simulink model "controller"  (Simulink 8.8)
settings: Solver=FixedStepDiscrete  StartTime=0.0  StopTime=inf  FixedStep=Ts  RelTol=1e-3  EnableMultiTasking=on
InitFcn:
  | clc
  | cd(fileparts(which(bdroot)));
  | initTrqBalancingSeeSaw;
undefined symbols (not defined in the file): bVectorConstraints, CONFIG, ConstraintsMatrix, directionOfOscillation, gain, LEFT_RIGHT_FOOT_IN_CONTACT, noOscillationTime, referenceParams, reg, ROBOT_DOF, sat, seesaw, WBT_robotName
libraries: WBToolboxLibrary x51, simulink x2
settings Model: SuppressorTable=22 serialization::archive 11 0 3 0 0 0 11 0  Creator=makaveli  LastModifiedBy=gnava
settings DataIOCC: SignalLoggingSaveFormat=Dataset
settings DebuggingCC: UnderspecifiedInitializationDetection=Simplified  MergeDetectMultiDrivingBlocksExec=error  SolverPrmCheckMsg=warning  FcnCallInpInsideContextMsg=error  AllowSymbolicDim=off  StateNameClashWarn=none
settings GRTTargetCC: CombineOutputUpdateFcns=on  GRTInterface=off
settings ConfigComp: CovSFcnEnable=off

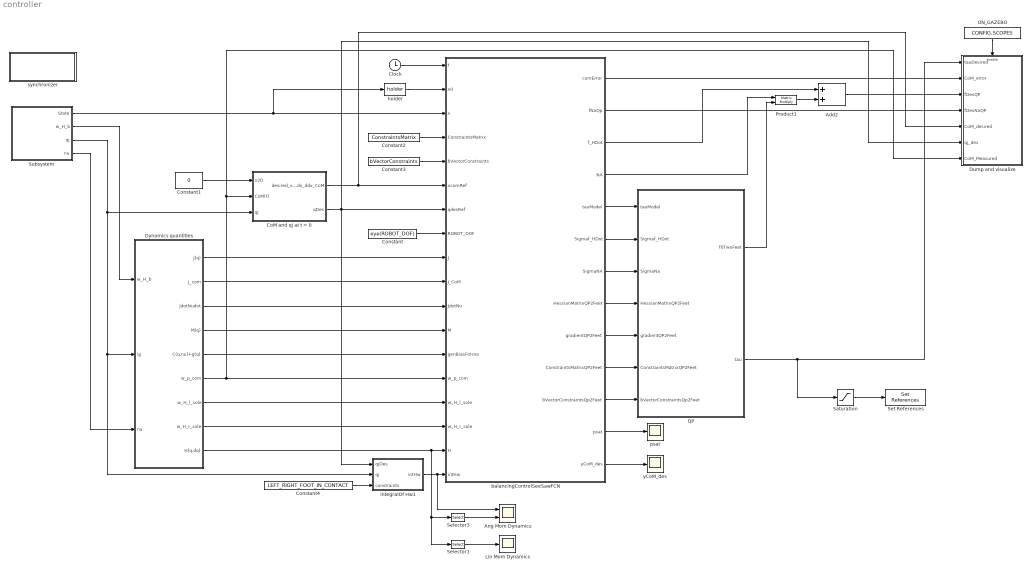
== system controller ==
  Add2 : Sum
  Ang Mom Dynamics : Scope  NumInputPorts=2
  Clock : Clock
  CoM and qj at t = 0 : Subsystem  Priority=2
  Constant : Constant  Value=eye(ROBOT_DOF)
  Constant1 : Constant  Value=0
  Constant2 : Constant  Value=ConstraintsMatrix
  Constant3 : Constant  Value=bVectorConstraints
  Constant4 : Constant  Value=LEFT_RIGHT_FOOT_IN_CONTACT
  Dump and visualize : Subsystem
  Dynamics quantities : Subsystem  Priority=3
  Lin Mom Dynamics : Scope
  "ON_GAZEBO " : Constant  Value=CONFIG.SCOPES
  Product1 : Product  Multiplication=Matrix(*)
  QP : Subsystem
  Saturation : Saturate  UpperLimit=sat.torque  LowerLimit=-sat.torque
  Selector1 : Selector  InputPortWidth=6  IndexOptions=Index vector (dialog)  Indices=[1 2 3]  OutputSizes=1
  Selector3 : Selector  InputPortWidth=6  IndexOptions=Index vector (dialog)  Indices=[4 5 6]  OutputSizes=1
  Set References : WBToolboxLibrary/wholeBodyActuators/Set References  controlType=Torque  fullOrSubControl=Full  controlledJoints=''  robotName=WBT_robotName  localName=WBT_modelName  wbiFile=WBT_wbiFilename  wbiList=WBT_wbiList
  Subsystem : Subsystem  Priority=1
      mask Display:
      | disp('State');
      | port_label('output',1,'x')
      | port_label('output',2,'w_H_b')
      | port_label('output',3,'q_j')
      | port_label('output',4,'nu')
  balancingControlSeeSawFCN : MATLAB Function  TreatAsAtomicUnit=on
  "holder " : WBToolboxLibrary/Utilities/holder 
  integralOf Hw1 : Subsystem
  psat : Scope
  synchronizer : Subsystem
      mask Display: disp('SYNCHRONIZER')
  yCoM_des : Scope
  wires:
  Clock/1 -> balancingControlSeeSawFCN/1(t)
  Subsystem/1(State) -> balancingControlSeeSawFCN/3(x), "holder "/1
  Subsystem/4(nu) -> Dynamics quantities/3(nu)
  CoM and qj at t = 0/2(qDes) -> integralOf Hw1/1(qjDes), Dump and visualize/6(qj_des), balancingControlSeeSawFCN/7(qdesRef)
  Constant/1 -> balancingControlSeeSawFCN/8(ROBOT_DOF)
  Dynamics quantities/1("J(q) ") -> balancingControlSeeSawFCN/9(J)
  Dynamics quantities/2(J_com) -> balancingControlSeeSawFCN/10(J_CoM)
  Dynamics quantities/3(JdotNudot) -> balancingControlSeeSawFCN/11(JdotNu)
  Dynamics quantities/4(M(q)) -> balancingControlSeeSawFCN/12(M)
  Dynamics quantities/5(C(q,nu)+g(q)) -> balancingControlSeeSawFCN/13(genBiasForces)
  Dynamics quantities/6(w_p_com) -> balancingControlSeeSawFCN/14(w_p_com), CoM and qj at t = 0/2(CoM(t)), Dump and visualize/7(CoM_Measured)
  Dynamics quantities/7(w_H_l_sole) -> balancingControlSeeSawFCN/15(w_H_l_sole)
  Dynamics quantities/8(w_H_r_sole) -> balancingControlSeeSawFCN/16(w_H_r_sole)
  Dynamics quantities/9(H(q,dq)) -> Selector1/1, Selector3/1, balancingControlSeeSawFCN/17(H)
  Saturation/1 -> Set References/1
  "holder "/1 -> balancingControlSeeSawFCN/2(x0)
  Subsystem/2(w_H_b) -> Dynamics quantities/1(w_H_b)
  Subsystem/3(qj) -> CoM and qj at t = 0/3(qj), integralOf Hw1/2(qj), Dynamics quantities/2(qj)
  Constant1/1 -> CoM and qj at t = 0/1(x2D)
  Constant2/1 -> balancingControlSeeSawFCN/4(ConstraintsMatrix)
  Constant3/1 -> balancingControlSeeSawFCN/5(bVectorConstraints)
  QP/1(f0TwoFeet) -> Product1/2
  QP/2(tau) -> Dump and visualize/1(tauDesired), Saturation/1
  "ON_GAZEBO "/1 -> Dump and visualize/Enable
  CoM and qj at t = 0/1(desired_x_dx_ddx_CoM) -> Dump and visualize/5(CoM_desired), balancingControlSeeSawFCN/6(xcomRef)
  balancingControlSeeSawFCN/1(comError) -> Dump and visualize/2(CoM_error)
  balancingControlSeeSawFCN/2(fNoQp) -> Dump and visualize/4(fDesNoQP)
  Product1/1 -> Add2/2
  balancingControlSeeSawFCN/4(NA) -> Product1/1
  balancingControlSeeSawFCN/3(f_HDot) -> Add2/1
  Add2/1 -> Dump and visualize/3(fDesQP)
  integralOf Hw1/1(intHw) -> Ang Mom Dynamics/1, balancingControlSeeSawFCN/18(intHw)
  balancingControlSeeSawFCN/5(tauModel) -> QP/1(tauModel)
  balancingControlSeeSawFCN/6(Sigmaf_HDot) -> QP/2(Sigmaf_HDot)
  balancingControlSeeSawFCN/7(SigmaNA) -> QP/3(SigmaNa)
  balancingControlSeeSawFCN/8(HessianMatrixQP2Feet) -> QP/4(HessianMatrixQP2Feet)
  balancingControlSeeSawFCN/9(gradientQP2Feet) -> QP/5(gradientQP2Feet)
  balancingControlSeeSawFCN/10(ConstraintsMatrixQP2Feet) -> QP/6(ConstraintsMatrixQP2Feet)
  balancingControlSeeSawFCN/11(bVectorConstraintsQp2Feet) -> QP/7(bVectorConstraintsQp2Feet)
  balancingControlSeeSawFCN/12(psat) -> psat/1
  balancingControlSeeSawFCN/13(yCoM_des) -> yCoM_des/1
  Constant4/1 -> integralOf Hw1/3(constraints)
  Selector3/1 -> Ang Mom Dynamics/2
  Selector1/1 -> Lin Mom Dynamics/1

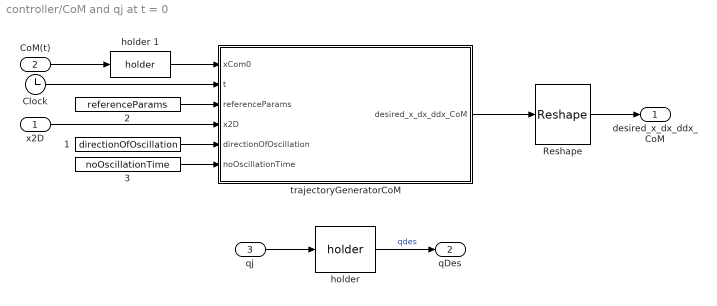
== system controller/CoM and qj at t = 0 ==
  x2D : Inport
  CoM(t) : Inport  Port=2
  qj : Inport  Port=3
  "    1" : Constant  Value=directionOfOscillation
  "    2" : Constant  Value=referenceParams
  "    3" : Constant  Value=noOscillationTime
  Clock : Clock
  Reshape : Reshape  OutputDimensionality=Customize  OutputDimensions=[3,3]
  "holder " : WBToolboxLibrary/Utilities/holder 
  holder 1 : WBToolboxLibrary/Utilities/holder 
  trajectoryGeneratorCoM : MATLAB Function  TreatAsAtomicUnit=on
  desired_x_dx_ddx_CoM : Outport
  qDes : Outport  Port=2
  wires:
  qj/1 -> "holder "/1
  "holder "/1 -> qDes/1  "qdes"
  holder 1/1 -> trajectoryGeneratorCoM/1(xCom0)
  "    2"/1 -> trajectoryGeneratorCoM/3(referenceParams)
  Clock/1 -> trajectoryGeneratorCoM/2(t)
  "    1"/1 -> trajectoryGeneratorCoM/5(directionOfOscillation)
  "    3"/1 -> trajectoryGeneratorCoM/6(noOscillationTime)
  trajectoryGeneratorCoM/1(desired_x_dx_ddx_CoM) -> Reshape/1
  Reshape/1 -> desired_x_dx_ddx_CoM/1
  x2D/1 -> trajectoryGeneratorCoM/4(x2D)
  CoM(t)/1 -> holder 1/1

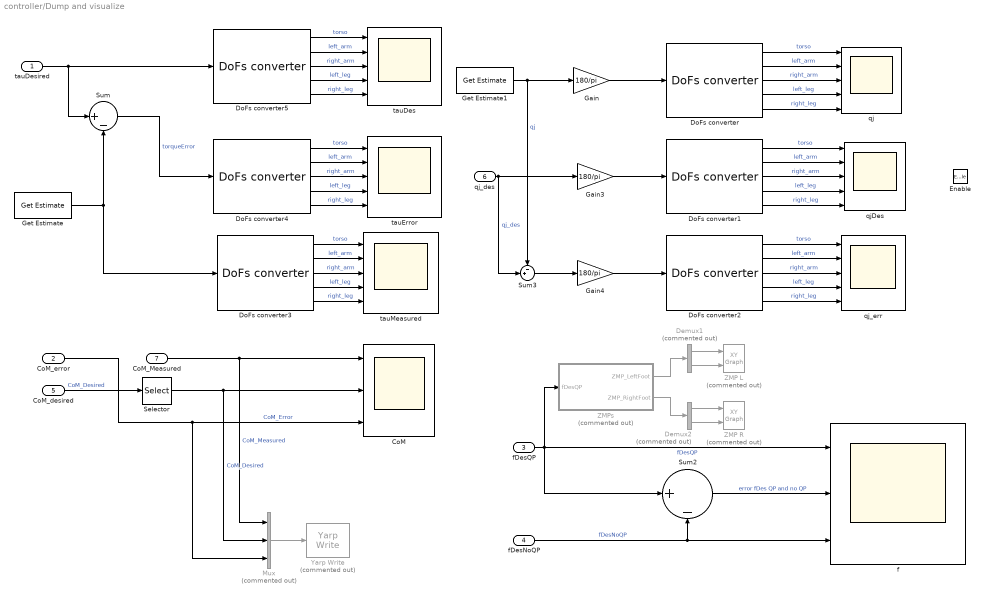
== system controller/Dump and visualize ==
  tauDesired : Inport
  CoM_error : Inport  Port=2
  fDesQP : Inport  Port=3
  fDesNoQP : Inport  Port=4
  CoM_desired : Inport  Port=5
  qj_des : Inport  Port=6
  CoM_Measured : Inport  Port=7
  Enable : EnablePort
  CoM : Scope  NumInputPorts=3
  Demux1 : Demux  Commented=on  Outputs=2
  Demux2 : Demux  Commented=on  Outputs=2
  DoFs converter{,1..5} (6 alike) : WBToolboxLibrary/Utilities/DoFs converter  yarp2WBIOption=From WBI to YARP  robotName=WBT_robotName  localName=WBT_modelName  wbiFile=WBT_wbiFilename  wbiList=WBT_wbiList
  Gain : Gain  Gain=180/pi
  Gain3 : Gain  Gain=180/pi
  Gain4 : Gain  Gain=180/pi
  Get Estimate : WBToolboxLibrary/wholeBodyStates/Get Estimate  estimateType=Joints Torque  robotName=WBT_robotName  localName=WBT_modelName  wbiFile=WBT_wbiFilename  wbiList=WBT_wbiList
  Get Estimate1 : WBToolboxLibrary/wholeBodyStates/Get Estimate  estimateType=Joints Position  robotName=WBT_robotName  localName=WBT_modelName  wbiFile=WBT_wbiFilename  wbiList=WBT_wbiList
  Mux : Mux  Commented=on  Inputs=3
  Selector : Selector  NumberOfDimensions=2  IndexOptions=Index vector (dialog),Index vector (dialog)  Indices=[1:3],1  OutputSizes=1,1
  Sum : Sum  Inputs=|+-
  Sum2 : Sum  Inputs=|+-
  Sum3 : Sum  Inputs=-+|
  Yarp Write : WBToolboxLibrary/Utilities/Yarp Write  Commented=on  portName='/oneFootBalancing/comInfo:o'  autoconnect=off  errorOnConnection=on
  ZMP L : simulink/Sinks/XY Graph  Commented=on  xmin=gain.footSize(1,1)  xmax=gain.footSize(1,2)  ymin=gain.footSize(2,1)  ymax=gain.footSize(2,2)  st=-1
  ZMP R : simulink/Sinks/XY Graph  Commented=on  xmin=gain.footSize(1,1)  xmax=gain.footSize(1,2)  ymin=gain.footSize(2,1)  ymax=gain.footSize(2,2)  st=-1
  ZMPs : Subsystem  Commented=on
  f : Scope  NumInputPorts=3
  qj : Scope  NumInputPorts=5
  qjDes : Scope  NumInputPorts=5
  qj_err : Scope  NumInputPorts=5
  tauDes : Scope  NumInputPorts=5
  tauError : Scope  NumInputPorts=5
  tauMeasured : Scope  NumInputPorts=5
  wires:
  CoM_error/1 -> Mux/3, CoM/3  "CoM_Error"
  CoM_desired/1 -> Selector/1  "CoM_Desired"
  CoM_Measured/1 -> Mux/1, CoM/1  "CoM_Measured"
  Get Estimate1/1 -> Sum3/1, Gain/1  "qj"
  Gain/1 -> DoFs converter/1
  DoFs converter/5 -> qj/5  "right_leg"
  DoFs converter/1 -> qj/1  "torso"
  DoFs converter/2 -> qj/2  "left_arm"
  DoFs converter/4 -> qj/4  "left_leg"
  DoFs converter/3 -> qj/3  "right_arm"
  fDesQP/1 -> ZMPs/1(fDesQP), Sum2/1, f/1  "fDesQP"
  ZMPs/1(ZMP_LeftFoot) -> Demux1/1
  ZMPs/2(ZMP_RightFoot) -> Demux2/1
  Demux1/1 -> ZMP L/1
  Demux1/2 -> ZMP L/2
  Demux2/1 -> ZMP R/1
  Demux2/2 -> ZMP R/2
  Sum2/1 -> f/2  "error fDes QP and no QP"
  fDesNoQP/1 -> Sum2/2, f/3  "fDesNoQP"
  tauDesired/1 -> DoFs converter5/1, Sum/1
  Get Estimate/1 -> DoFs converter3/1, Sum/2
  DoFs converter5/5 -> tauDes/5  "right_leg"
  DoFs converter5/1 -> tauDes/1  "torso"
  DoFs converter5/2 -> tauDes/2  "left_arm"
  DoFs converter5/4 -> tauDes/4  "left_leg"
  DoFs converter5/3 -> tauDes/3  "right_arm"
  DoFs converter4/5 -> tauError/5  "right_leg"
  DoFs converter4/1 -> tauError/1  "torso"
  DoFs converter4/2 -> tauError/2  "left_arm"
  DoFs converter4/4 -> tauError/4  "left_leg"
  DoFs converter4/3 -> tauError/3  "right_arm"
  Sum/1 -> DoFs converter4/1  "torqueError"
  DoFs converter3/5 -> tauMeasured/5  "right_leg"
  DoFs converter3/1 -> tauMeasured/1  "torso"
  DoFs converter3/2 -> tauMeasured/2  "left_arm"
  DoFs converter3/4 -> tauMeasured/4  "left_leg"
  DoFs converter3/3 -> tauMeasured/3  "right_arm"
  qj_des/1 -> Sum3/2, Gain3/1  "qj_des"
  Gain3/1 -> DoFs converter1/1
  DoFs converter1/5 -> qjDes/5  "right_leg"
  DoFs converter1/1 -> qjDes/1  "torso"
  DoFs converter1/2 -> qjDes/2  "left_arm"
  DoFs converter1/4 -> qjDes/4  "left_leg"
  DoFs converter1/3 -> qjDes/3  "right_arm"
  Gain4/1 -> DoFs converter2/1
  DoFs converter2/5 -> qj_err/5  "right_leg"
  DoFs converter2/1 -> qj_err/1  "torso"
  DoFs converter2/2 -> qj_err/2  "left_arm"
  DoFs converter2/4 -> qj_err/4  "left_leg"
  DoFs converter2/3 -> qj_err/3  "right_arm"
  Sum3/1 -> Gain4/1
  Selector/1 -> Mux/2, CoM/2  "CoM_Desired"
  Mux/1 -> Yarp Write/1

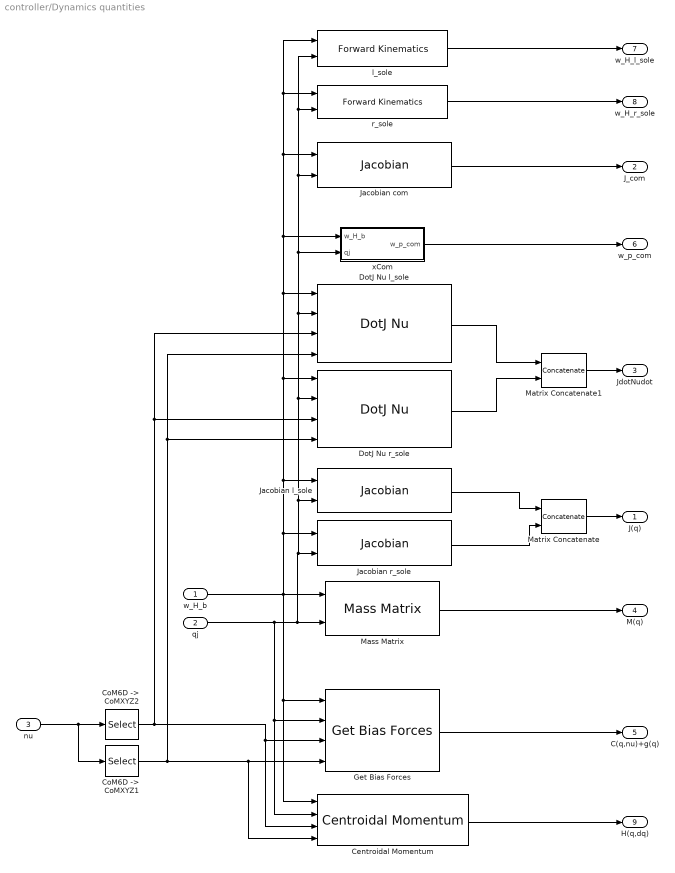
== system controller/Dynamics quantities ==
  w_H_b : Inport
  qj : Inport  Port=2
  nu : Inport  Port=3
  Centroidal Momentum : WBToolboxLibrary/wholeBodyModel/Dynamics/Centroidal Momentum  robotName=WBT_robotName  localName=WBT_modelName  wbiFile=WBT_wbiFilename  wbiList=WBT_wbiList
  "CoM6D ->  CoMXYZ1" : Selector  InputPortWidth=6+ROBOT_DOF  IndexOptions=Index vector (dialog)  Indices=[7:6+ROBOT_DOF]  OutputSizes=1
  "CoM6D ->  CoMXYZ2" : Selector  InputPortWidth=6+ROBOT_DOF  IndexOptions=Index vector (dialog)  Indices=[1 2 3 4 5 6]  OutputSizes=1
  "DotJ Nu l_sole " : WBToolboxLibrary/wholeBodyModel/Jacobians/DotJ Nu  frameName='l_sole'  robotName=WBT_robotName  localName=WBT_modelName  wbiFile=WBT_wbiFilename  wbiList=WBT_wbiList
  "DotJ Nu r_sole " : WBToolboxLibrary/wholeBodyModel/Jacobians/DotJ Nu  frameName='r_sole'  robotName=WBT_robotName  localName=WBT_modelName  wbiFile=WBT_wbiFilename  wbiList=WBT_wbiList
  Get Bias Forces : WBToolboxLibrary/wholeBodyModel/Dynamics/Get Bias Forces  robotName=WBT_robotName  localName=WBT_modelName  wbiFile=WBT_wbiFilename  wbiList=WBT_wbiList  explicitGravity=off
  Jacobian com : WBToolboxLibrary/wholeBodyModel/Jacobians/Jacobian  frameName='com'  robotName=WBT_robotName  localName=WBT_modelName  wbiFile=WBT_wbiFilename  wbiList=WBT_wbiList
  Jacobian l_sole : WBToolboxLibrary/wholeBodyModel/Jacobians/Jacobian  frameName='l_sole'  robotName=WBT_robotName  localName=WBT_modelName  wbiFile=WBT_wbiFilename  wbiList=WBT_wbiList
  Jacobian r_sole : WBToolboxLibrary/wholeBodyModel/Jacobians/Jacobian  frameName='r_sole'  robotName=WBT_robotName  localName=WBT_modelName  wbiFile=WBT_wbiFilename  wbiList=WBT_wbiList
  Mass Matrix : WBToolboxLibrary/wholeBodyModel/Dynamics/Mass Matrix  robotName=WBT_robotName  localName=WBT_modelName  wbiFile=WBT_wbiFilename  wbiList=WBT_wbiList
  Matrix Concatenate : Concatenate  Mode=Multidimensional array
  Matrix Concatenate1 : Concatenate  Mode=Multidimensional array
  l_sole : WBToolboxLibrary/wholeBodyModel/Kinematics/Forward Kinematics  frameName='l_sole'  robotName=WBT_robotName  localName=WBT_modelName  wbiFile=WBT_wbiFilename  wbiList=WBT_wbiList
  r_sole : WBToolboxLibrary/wholeBodyModel/Kinematics/Forward Kinematics  frameName='r_sole'  robotName=WBT_robotName  localName=WBT_modelName  wbiFile=WBT_wbiFilename  wbiList=WBT_wbiList
  xCom : Subsystem
  "J(q) " : Outport
  J_com : Outport  Port=2
  JdotNudot : Outport  Port=3
  M(q) : Outport  Port=4
  C(q,nu)+g(q) : Outport  Port=5
  w_p_com : Outport  Port=6
  w_H_l_sole : Outport  Port=7
  w_H_r_sole : Outport  Port=8
  H(q,dq) : Outport  Port=9
  wires:
  Get Bias Forces/1 -> C(q,nu)+g(q)/1
  Matrix Concatenate1/1 -> JdotNudot/1
  Jacobian r_sole/1 -> Matrix Concatenate/2
  l_sole/1 -> w_H_l_sole/1
  xCom/1(w_p_com) -> w_p_com/1
  r_sole/1 -> w_H_r_sole/1
  Matrix Concatenate/1 -> "J(q) "/1
  Jacobian l_sole/1 -> Matrix Concatenate/1
  Jacobian com/1 -> J_com/1
  w_H_b/1 -> Jacobian r_sole/1, "DotJ Nu r_sole "/1, r_sole/1, l_sole/1, Jacobian com/1, xCom/1(w_H_b), "DotJ Nu l_sole "/1, Jacobian l_sole/1, Mass Matrix/1, Centroidal Momentum/1, Get Bias Forces/1
  qj/1 -> r_sole/2, l_sole/2, Jacobian com/2, xCom/2(qj), "DotJ Nu l_sole "/2, "DotJ Nu r_sole "/2, Jacobian l_sole/2, Jacobian r_sole/2, Mass Matrix/2, Get Bias Forces/2, Centroidal Momentum/2
  "CoM6D ->  CoMXYZ2"/1 -> "DotJ Nu r_sole "/3, "DotJ Nu l_sole "/3, Centroidal Momentum/3, Get Bias Forces/3
  "CoM6D ->  CoMXYZ1"/1 -> "DotJ Nu r_sole "/4, "DotJ Nu l_sole "/4, Get Bias Forces/4, Centroidal Momentum/4
  nu/1 -> "CoM6D ->  CoMXYZ1"/1, "CoM6D ->  CoMXYZ2"/1
  Centroidal Momentum/1 -> H(q,dq)/1
  Mass Matrix/1 -> M(q)/1
  "DotJ Nu l_sole "/1 -> Matrix Concatenate1/1
  "DotJ Nu r_sole "/1 -> Matrix Concatenate1/2

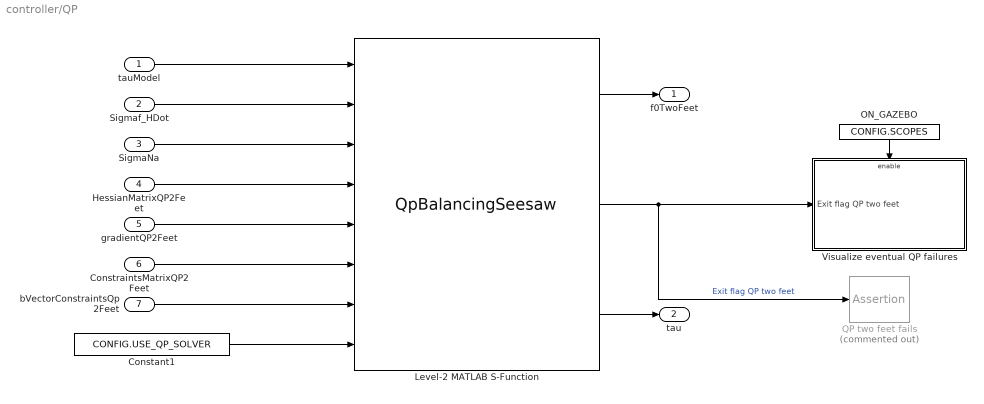
== system controller/QP ==
  tauModel : Inport
  Sigmaf_HDot : Inport  Port=2
  SigmaNa : Inport  Port=3
  HessianMatrixQP2Feet : Inport  Port=4
  gradientQP2Feet : Inport  Port=5
  ConstraintsMatrixQP2Feet : Inport  Port=6
  bVectorConstraintsQp2Feet : Inport  Port=7
  Constant1 : Constant  Value=CONFIG.USE_QP_SOLVER
  Level-2 MATLAB S-Function : M-S-Function  FunctionName=QpBalancingSeesaw
  "ON_GAZEBO " : Constant  Value=CONFIG.SCOPES
  QP two feet fails : Assertion  Commented=on
  Visualize eventual QP failures : Subsystem
  f0TwoFeet : Outport
  tau : Outport  Port=2
  wires:
  Level-2 MATLAB S-Function/1 -> f0TwoFeet/1
  Level-2 MATLAB S-Function/2 -> QP two feet fails/1, Visualize eventual QP failures/1(Exit flag QP two feet)  "Exit flag QP two feet"
  "ON_GAZEBO "/1 -> Visualize eventual QP failures/Enable
  Constant1/1 -> Level-2 MATLAB S-Function/8
  HessianMatrixQP2Feet/1 -> Level-2 MATLAB S-Function/4
  gradientQP2Feet/1 -> Level-2 MATLAB S-Function/5
  ConstraintsMatrixQP2Feet/1 -> Level-2 MATLAB S-Function/6
  bVectorConstraintsQp2Feet/1 -> Level-2 MATLAB S-Function/7
  tauModel/1 -> Level-2 MATLAB S-Function/1
  Sigmaf_HDot/1 -> Level-2 MATLAB S-Function/2
  SigmaNa/1 -> Level-2 MATLAB S-Function/3
  Level-2 MATLAB S-Function/3 -> tau/1

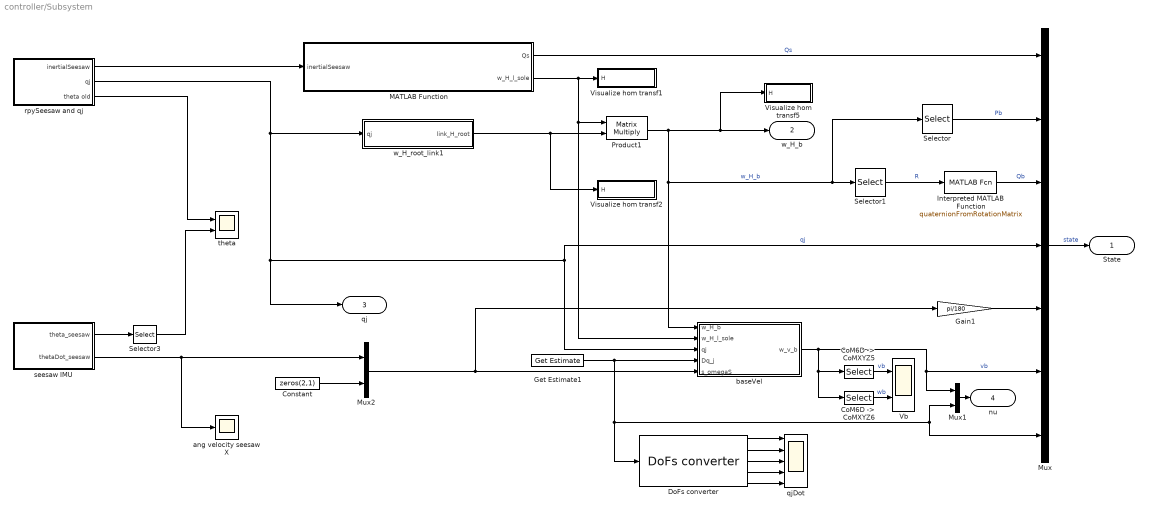
== system controller/Subsystem ==
  "CoM6D ->  CoMXYZ5" : Selector  InputPortWidth=6  IndexOptions=Index vector (dialog)  Indices=[1 2 3]  OutputSizes=1
  "CoM6D ->  CoMXYZ6" : Selector  InputPortWidth=6  IndexOptions=Index vector (dialog)  Indices=[4 5 6]  OutputSizes=1
  Constant : Constant  Value=zeros(2,1)
  DoFs converter : WBToolboxLibrary/Utilities/DoFs converter  yarp2WBIOption=From WBI to YARP  robotName=WBT_robotName  localName=WBT_modelName  wbiFile=WBT_wbiFilename  wbiList=WBT_wbiList
  Gain1 : Gain  Gain=pi/180
  Get Estimate1 : WBToolboxLibrary/wholeBodyStates/Get Estimate  estimateType=Joints Velocity  robotName=WBT_robotName  localName=WBT_modelName  wbiFile=WBT_wbiFilename  wbiList=WBT_wbiList
  Interpreted MATLAB Function : MATLABFcn  MATLABFcn=quaternionFromRotationMatrix  OutputDimensions=4
  MATLAB Function : MATLAB Function  Priority=10  TreatAsAtomicUnit=on
  Mux : Mux  Inputs=7
  Mux1 : Mux  Inputs=2
  Mux2 : Mux  Inputs=2
  Product1 : Product  Priority=19  Multiplication=Matrix(*)
  Selector : Selector  NumberOfDimensions=2  InputPortWidth=3  IndexOptions=Index vector (dialog),Index vector (dialog)  Indices=[1:3],4  OutputSizes=1,1
  Selector1 : Selector  NumberOfDimensions=2  InputPortWidth=3  IndexOptions=Index vector (dialog),Index vector (dialog)  Indices=[1:3],[1:3]  OutputSizes=1,1
  Selector3 : Selector  InputPortWidth=3  IndexOptions=Index vector (dialog)  Indices=[1]  OutputSizes=1
  "Vb " : Scope  NumInputPorts=2
  Visualize hom transf1 : Subsystem
  Visualize hom transf2 : Subsystem
  Visualize hom transf5 : Subsystem
  ang velocity seesaw X : Scope
  baseVel : Subsystem
  qjDot : Scope  NumInputPorts=5
  rpySeesaw and qj : Subsystem
  seesaw IMU : Subsystem
  theta : Scope  NumInputPorts=2
  w_H_root_link1 : Subsystem  mask{link_name='l_sole'}
      mask prompts: link_name "link name"
      mask help:
      | This block evaluates the homogeneous transformation between the world and the root link, i.e. ^wH_b. It assumes that the link specified by the variable 'link_name' has a constant position
      | w.r.t. an inertial frame, but it can rotate arbitrarily. This rotation is retrived from the IMU sensor.
      mask Display:
      | str = strrep(link_name, '_','\_');
      | port_label('output',1,['{}^{',str '}H_{root}'],'texmode','on')
      | clear str;
      | 
      | port_label('input',1,'q_j','texmode','on')
  State : Outport
  w_H_b : Outport  Port=2
  qj : Outport  Port=3
  nu : Outport  Port=4
  wires:
  Get Estimate1/1 -> baseVel/4(Dq_j), DoFs converter/1, Mux1/2, Mux/7
  rpySeesaw and qj/2(qj) -> w_H_root_link1/1(qj), qj/1, baseVel/3(qj), Mux/4  "qj"
  Mux/1 -> State/1  "state"
  Selector/1 -> Mux/2  "Pb"
  Selector1/1 -> Interpreted MATLAB Function/1  "R"
  Interpreted MATLAB Function/1 -> Mux/3  "Qb"
  Mux1/1 -> nu/1
  baseVel/1(w_v_b) -> Mux1/1, Mux/6, "CoM6D ->  CoMXYZ5"/1, "CoM6D ->  CoMXYZ6"/1  "vb"
  MATLAB Function/1(Qs) -> Mux/1  "Qs"
  Product1/1 -> Visualize hom transf5/1(H), w_H_b/1, baseVel/1(w_H_b), Selector1/1, Selector/1  "w_H_b"
  MATLAB Function/2(w_H_l_sole) -> baseVel/2(w_H_l_sole), Product1/1, Visualize hom transf1/1(H)
  w_H_root_link1/1(link_H_root) -> Visualize hom transf2/1(H), Product1/2
  DoFs converter/1 -> qjDot/1
  DoFs converter/2 -> qjDot/2
  DoFs converter/3 -> qjDot/3
  DoFs converter/4 -> qjDot/4
  DoFs converter/5 -> qjDot/5
  "CoM6D ->  CoMXYZ5"/1 -> "Vb "/1  "vb"
  "CoM6D ->  CoMXYZ6"/1 -> "Vb "/2  "wb"
  Gain1/1 -> Mux/5
  Mux2/1 -> Gain1/1, baseVel/5(s_omegaS)
  Constant/1 -> Mux2/2
  rpySeesaw and qj/1(inertialSeesaw) -> MATLAB Function/1(inertialSeesaw)
  rpySeesaw and qj/3(theta old) -> theta/1
  seesaw IMU/2(thetaDot_seesaw) -> Mux2/1, ang velocity seesaw X/1
  seesaw IMU/1(theta_seesaw) -> Selector3/1
  Selector3/1 -> theta/2

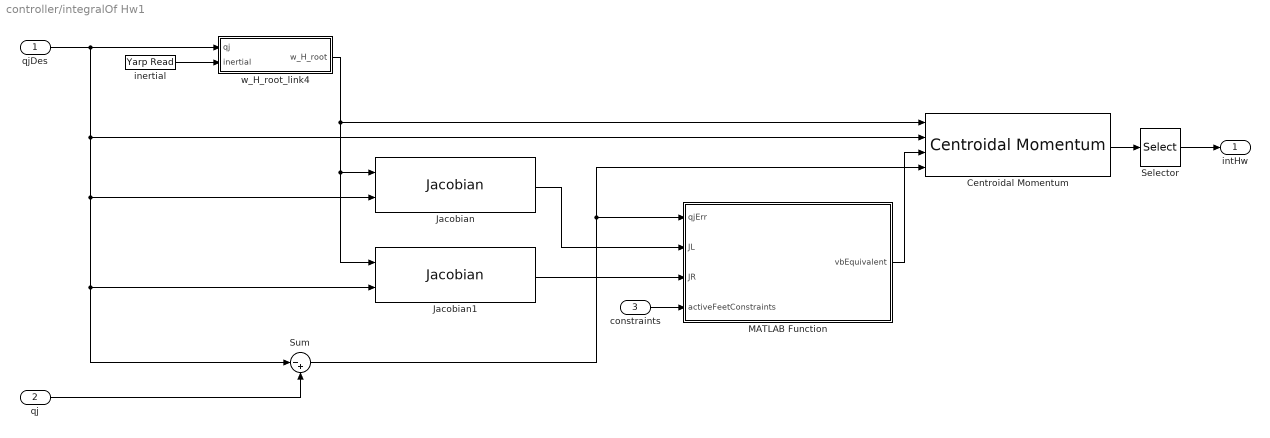
== system controller/integralOf Hw1 ==
  qjDes : Inport
  qj : Inport  Port=2
  constraints : Inport  Port=3
  Centroidal Momentum : WBToolboxLibrary/wholeBodyModel/Dynamics/Centroidal Momentum  robotName=WBT_robotName  localName=WBT_modelName  wbiFile=WBT_wbiFilename  wbiList=WBT_wbiList
  Jacobian : WBToolboxLibrary/wholeBodyModel/Jacobians/Jacobian  frameName='l_sole'  robotName=WBT_robotName  localName=WBT_modelName  wbiFile=WBT_wbiFilename  wbiList=WBT_wbiList
  Jacobian1 : WBToolboxLibrary/wholeBodyModel/Jacobians/Jacobian  frameName='r_sole'  robotName=WBT_robotName  localName=WBT_modelName  wbiFile=WBT_wbiFilename  wbiList=WBT_wbiList
  MATLAB Function : MATLAB Function  TreatAsAtomicUnit=on
  Selector : Selector  InputPortWidth=6  IndexOptions=Index vector (dialog)  Indices=[4 5 6]  OutputSizes=1
  Sum : Sum  Inputs=|-+
  inertial : WBToolboxLibrary/Utilities/Yarp Read  portName=PORTS.IMU  signalSize=12  blocking=off  timestamp=off  autoconnect=on  errorOnConnection=on
  w_H_root_link4 : Subsystem  mask{link_name='l_sole'}
      mask prompts: link_name "link name"
      mask help:
      | This block evaluates the homogeneous transformation between the world and the root link, i.e. ^wH_b. It assumes that the link specified by the variable 'link_name' has a constant position
      | w.r.t. an inertial frame, but it can rotate arbitrarily. This rotation is retrived from the IMU sensor.
      mask Display:
      | str = strrep(link_name, '_','\_');
      | port_label('output',1,['{}^{',str '}H_{root}'],'texmode','on')
      | clear str;
      | 
      | port_label('input',1,'q_j','texmode','on')
      | 
      | port_label('input',2,'inertial','texmode','on')
  intHw : Outport
  wires:
  qjDes/1 -> Sum/1, Jacobian1/2, Jacobian/2, Centroidal Momentum/2, w_H_root_link4/1(qj)
  w_H_root_link4/1(w_H_root) -> Centroidal Momentum/1, Jacobian/1, Jacobian1/1
  qj/1 -> Sum/2
  Sum/1 -> Centroidal Momentum/4, MATLAB Function/1(qjErr)
  MATLAB Function/1(vbEquivalent) -> Centroidal Momentum/3
  Jacobian/1 -> MATLAB Function/2(JL)
  Centroidal Momentum/1 -> Selector/1
  Selector/1 -> intHw/1
  Jacobian1/1 -> MATLAB Function/3(JR)
  constraints/1 -> MATLAB Function/4(activeFeetConstraints)
  inertial/1 -> w_H_root_link4/2(inertial)

== system controller/synchronizer ==
  GAZEBO_SYNCHRONIZER : Subsystem  Commented=on
  Logical Operator : Logic  Operator=NOT  AllPortsSameDT=off  OutDataTypeStr=boolean
  "ON_GAZEBO " : Constant  Value=CONFIG.ON_GAZEBO
  REAL_TIME_SYNC : Subsystem
  wires:
  Logical Operator/1 -> REAL_TIME_SYNC/Enable
  "ON_GAZEBO "/1 -> Logical Operator/1, GAZEBO_SYNCHRONIZER/Enable

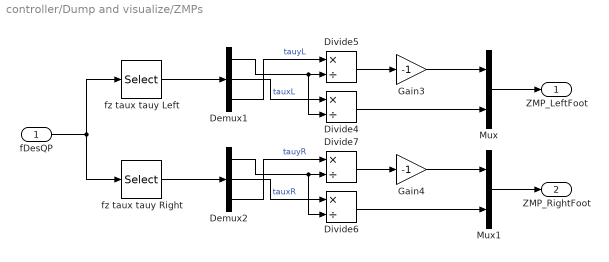
== system controller/Dump and visualize/ZMPs ==
  fDesQP : Inport
  Demux1 : Demux  Outputs=3
  Demux2 : Demux  Outputs=3
  Divide{4..7} (4 alike) : Product  Inputs=*/
  Gain3 : Gain  Gain=-1
  Gain4 : Gain  Gain=-1
  Mux : Mux  Inputs=2
  Mux1 : Mux  Inputs=2
  fz taux tauy Left : Selector  InputPortWidth=12  IndexOptions=Index vector (dialog)  Indices=[3 4 5]  OutputSizes=1
  fz taux tauy Right : Selector  InputPortWidth=12  IndexOptions=Index vector (dialog)  Indices=[9 10 11]  OutputSizes=1
  ZMP_LeftFoot : Outport
  ZMP_RightFoot : Outport  Port=2
  wires:
  fz taux tauy Left/1 -> Demux1/1
  Demux1/1 -> Divide4/2, Divide5/2
  Divide7/1 -> Gain4/1
  Divide4/1 -> Mux/2
  Divide5/1 -> Gain3/1
  fz taux tauy Right/1 -> Demux2/1
  Demux2/1 -> Divide6/2, Divide7/2
  fDesQP/1 -> fz taux tauy Left/1, fz taux tauy Right/1
  Gain3/1 -> Mux/1
  Mux/1 -> ZMP_LeftFoot/1
  Divide6/1 -> Mux1/2
  Gain4/1 -> Mux1/1
  Mux1/1 -> ZMP_RightFoot/1
  Demux1/2 -> Divide4/1  "tauxL"
  Demux1/3 -> Divide5/1  "tauyL"
  Demux2/2 -> Divide6/1  "tauxR"
  Demux2/3 -> Divide7/1  "tauyR"

== system controller/Dynamics quantities/xCom ==
  w_H_b : Inport
  qj : Inport  Port=2
  "CoM6D ->  CoMXYZ2" : Selector  NumberOfDimensions=2  InputPortWidth=7  IndexOptions=Index vector (dialog),Index vector (dialog)  Indices=[1 2 3],[4]  OutputSizes=1,1
  com : WBToolboxLibrary/wholeBodyModel/Kinematics/Forward Kinematics  frameName='com'  robotName=WBT_robotName  localName=WBT_modelName  wbiFile=WBT_wbiFilename  wbiList=WBT_wbiList
  w_p_com : Outport
  wires:
  qj/1 -> com/2
  "CoM6D ->  CoMXYZ2"/1 -> w_p_com/1
  com/1 -> "CoM6D ->  CoMXYZ2"/1
  w_H_b/1 -> com/1

== system controller/QP/Visualize eventual QP failures ==
  Exit flag QP two feet : Inport
  Enable : EnablePort
  "QP status (0: no failure, 1: not using)" : Scope
  wires:
  Exit flag QP two feet/1 -> "QP status (0: no failure, 1: not using)"/1  "Exit flag QP two feet"

== system controller/Subsystem/Visualize hom transf1 ==
  H : Inport
  "CoM6D ->  CoMXYZ1" : Selector  NumberOfDimensions=2  InputPortWidth=7  IndexOptions=Index vector (dialog),Index vector (dialog)  Indices=[1 2 3],[1 2 3]  OutputSizes=1,1
  Hom : Scope
  MATLAB Function : MATLAB Function  TreatAsAtomicUnit=on
  p : Scope
  position : Selector  NumberOfDimensions=2  InputPortWidth=7  IndexOptions=Index vector (dialog),Index vector (dialog)  Indices=[1 2 3],[4]  OutputSizes=1,1
  rollPitchYaw : Scope
  wires:
  position/1 -> p/1  "position"
  H/1 -> position/1, Hom/1, "CoM6D ->  CoMXYZ1"/1  "H"
  "CoM6D ->  CoMXYZ1"/1 -> MATLAB Function/1(R)
  MATLAB Function/1(rollPitchYaw) -> rollPitchYaw/1  "rollPitchYaw"

== system controller/Subsystem/Visualize hom transf2 ==
  H : Inport
  "CoM6D ->  CoMXYZ1" : Selector  NumberOfDimensions=2  InputPortWidth=7  IndexOptions=Index vector (dialog),Index vector (dialog)  Indices=[1 2 3],[1 2 3]  OutputSizes=1,1
  Hom : Scope
  MATLAB Function : MATLAB Function  TreatAsAtomicUnit=on
  p : Scope
  position : Selector  NumberOfDimensions=2  InputPortWidth=7  IndexOptions=Index vector (dialog),Index vector (dialog)  Indices=[1 2 3],[4]  OutputSizes=1,1
  rollPitchYaw : Scope
  wires:
  position/1 -> p/1  "position"
  H/1 -> position/1, Hom/1, "CoM6D ->  CoMXYZ1"/1  "H"
  "CoM6D ->  CoMXYZ1"/1 -> MATLAB Function/1(R)
  MATLAB Function/1(rollPitchYaw) -> rollPitchYaw/1  "rollPitchYaw"

== system controller/Subsystem/Visualize hom transf5 ==
  H : Inport
  "CoM6D ->  CoMXYZ1" : Selector  NumberOfDimensions=2  InputPortWidth=7  IndexOptions=Index vector (dialog),Index vector (dialog)  Indices=[1 2 3],[1 2 3]  OutputSizes=1,1
  Hom : Scope
  MATLAB Function : MATLAB Function  TreatAsAtomicUnit=on
  p : Scope
  position : Selector  NumberOfDimensions=2  InputPortWidth=7  IndexOptions=Index vector (dialog),Index vector (dialog)  Indices=[1 2 3],[4]  OutputSizes=1,1
  rollPitchYaw : Scope
  wires:
  position/1 -> p/1  "position"
  H/1 -> position/1, Hom/1, "CoM6D ->  CoMXYZ1"/1  "H"
  "CoM6D ->  CoMXYZ1"/1 -> MATLAB Function/1(R)
  MATLAB Function/1(rollPitchYaw) -> rollPitchYaw/1  "rollPitchYaw"

== system controller/Subsystem/baseVel ==
  w_H_b : Inport
  w_H_l_sole : Inport  Port=2
  qj : Inport  Port=3
  Dq_j : Inport  Port=4
  s_omegaS : Inport  Port=5
  Jacobian l_sole : WBToolboxLibrary/wholeBodyModel/Jacobians/Jacobian  frameName='l_sole'  robotName=WBT_robotName  localName=WBT_modelName  wbiFile=WBT_wbiFilename  wbiList=WBT_wbiList
  evaluateBaseVelocity : MATLAB Function  Priority=10  TreatAsAtomicUnit=on
  w_v_b : Outport
  wires:
  w_H_l_sole/1 -> evaluateBaseVelocity/2(w_H_l_sole)
  w_H_b/1 -> Jacobian l_sole/1
  evaluateBaseVelocity/1(w_v_base) -> w_v_b/1
  s_omegaS/1 -> evaluateBaseVelocity/4(s_omega_s)
  qj/1 -> Jacobian l_sole/2
  Dq_j/1 -> evaluateBaseVelocity/3(dq_j)
  Jacobian l_sole/1 -> evaluateBaseVelocity/1(J_l_sole)

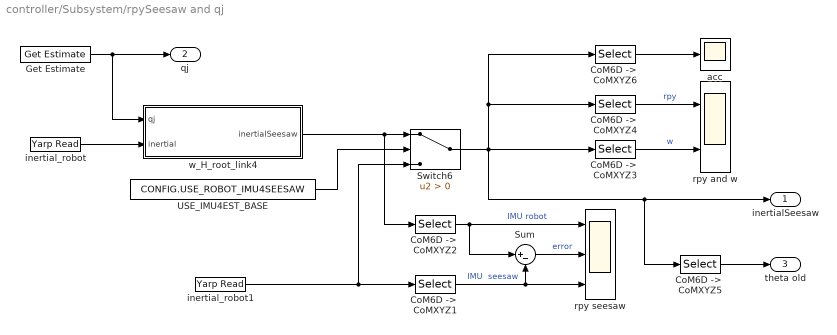
== system controller/Subsystem/rpySeesaw and qj ==
  "CoM6D ->  CoMXYZ1" : Selector  InputPortWidth=12  IndexOptions=Index vector (dialog)  Indices=[1 2 3]  OutputSizes=1
  "CoM6D ->  CoMXYZ2" : Selector  InputPortWidth=12  IndexOptions=Index vector (dialog)  Indices=[1 2 3]  OutputSizes=1
  "CoM6D ->  CoMXYZ3" : Selector  InputPortWidth=12  IndexOptions=Index vector (dialog)  Indices=[7 8 9]  OutputSizes=1
  "CoM6D ->  CoMXYZ4" : Selector  InputPortWidth=12  IndexOptions=Index vector (dialog)  Indices=[1 2 3]  OutputSizes=1
  "CoM6D ->  CoMXYZ5" : Selector  InputPortWidth=12  IndexOptions=Index vector (dialog)  Indices=[1]  OutputSizes=1
  "CoM6D ->  CoMXYZ6" : Selector  InputPortWidth=12  IndexOptions=Index vector (dialog)  Indices=[4 5 6]  OutputSizes=1
  Get Estimate : WBToolboxLibrary/wholeBodyStates/Get Estimate  estimateType=Joints Position  robotName=WBT_robotName  localName=WBT_modelName  wbiFile=WBT_wbiFilename  wbiList=WBT_wbiList
  Sum : Sum  Inputs=|+-
  Switch6 : Switch  Criteria=u2 > Threshold
  USE_IMU4EST_BASE : Constant  Value=CONFIG.USE_ROBOT_IMU4SEESAW
  acc : Scope
  inertial_robot : WBToolboxLibrary/Utilities/Yarp Read  portName=PORTS.IMU  signalSize=12  blocking=off  timestamp=off  autoconnect=on  errorOnConnection=on
  inertial_robot1 : WBToolboxLibrary/Utilities/Yarp Read  portName=PORTS.IMU  signalSize=12  blocking=off  timestamp=off  autoconnect=on  errorOnConnection=on
  rpy and w : Scope  NumInputPorts=2
  rpy seesaw : Scope  NumInputPorts=3
  w_H_root_link4 : Subsystem  mask{link_name='l_sole'}
      mask prompts: link_name "link name"
      mask help:
      | This block evaluates the homogeneous transformation between the world and the root link, i.e. ^wH_b. It assumes that the link specified by the variable 'link_name' has a constant position
      | w.r.t. an inertial frame, but it can rotate arbitrarily. This rotation is retrived from the IMU sensor.
      mask Display:
      | str = strrep(link_name, '_','\_');
      | port_label('output',1,'inertialSeesaw','texmode','on')
      | clear str;
      | 
      | port_label('input',1,'q_j','texmode','on')
      | 
      | port_label('input',2,'inertial','texmode','on')
  inertialSeesaw : Outport
  qj : Outport  Port=2
  theta old : Outport  Port=3
  wires:
  USE_IMU4EST_BASE/1 -> Switch6/2
  w_H_root_link4/1(inertialSeesaw) -> "CoM6D ->  CoMXYZ2"/1, Switch6/1
  Get Estimate/1 -> qj/1, w_H_root_link4/1(qj)
  inertial_robot/1 -> w_H_root_link4/2(inertial)
  "CoM6D ->  CoMXYZ2"/1 -> Sum/1, rpy seesaw/1  "IMU robot"
  Sum/1 -> rpy seesaw/2  "error"
  "CoM6D ->  CoMXYZ1"/1 -> Sum/2, rpy seesaw/3  "IMU  seesaw"
  "CoM6D ->  CoMXYZ3"/1 -> rpy and w/2  "w"
  "CoM6D ->  CoMXYZ4"/1 -> rpy and w/1  "rpy"
  "CoM6D ->  CoMXYZ5"/1 -> theta old/1
  inertial_robot1/1 -> Switch6/3, "CoM6D ->  CoMXYZ1"/1
  Switch6/1 -> "CoM6D ->  CoMXYZ6"/1, "CoM6D ->  CoMXYZ4"/1, "CoM6D ->  CoMXYZ3"/1, "CoM6D ->  CoMXYZ5"/1, inertialSeesaw/1
  "CoM6D ->  CoMXYZ6"/1 -> acc/1

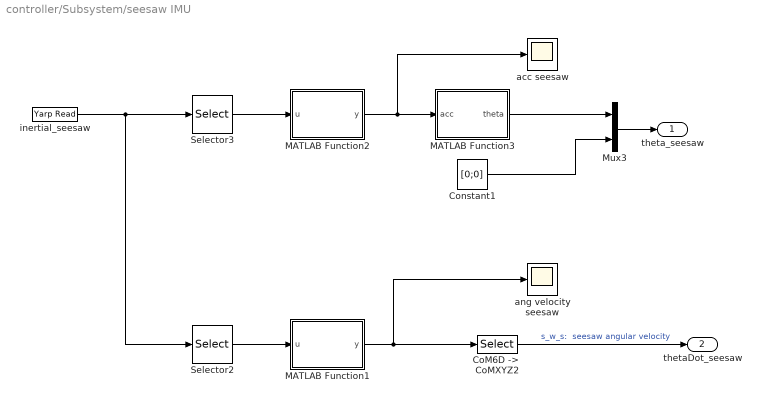
== system controller/Subsystem/seesaw IMU ==
  "CoM6D ->  CoMXYZ2" : Selector  InputPortWidth=3  IndexOptions=Index vector (dialog)  Indices=[1]  OutputSizes=1
  Constant1 : Constant  Value=[0;0]
  MATLAB Function1 : MATLAB Function  TreatAsAtomicUnit=on
  MATLAB Function2 : MATLAB Function  TreatAsAtomicUnit=on
  MATLAB Function3 : MATLAB Function  TreatAsAtomicUnit=on
  Mux3 : Mux  Inputs=2
  Selector2 : Selector  InputPortWidth=9  IndexOptions=Index vector (dialog)  Indices=[7 8 9]  OutputSizes=1
  Selector3 : Selector  InputPortWidth=9  IndexOptions=Index vector (dialog)  Indices=[4 5 6]  OutputSizes=1
  acc seesaw : Scope
  ang velocity seesaw : Scope
  inertial_seesaw : WBToolboxLibrary/Utilities/Yarp Read  portName='/seesaw'  signalSize=9  blocking=off  timestamp=off  autoconnect=on  errorOnConnection=on
  theta_seesaw : Outport
  thetaDot_seesaw : Outport  Port=2
  wires:
  Constant1/1 -> Mux3/2
  "CoM6D ->  CoMXYZ2"/1 -> thetaDot_seesaw/1  "s_w_s:  seesaw angular velocity"
  MATLAB Function2/1(y) -> acc seesaw/1, MATLAB Function3/1(acc)
  Selector3/1 -> MATLAB Function2/1(u)
  Selector2/1 -> MATLAB Function1/1(u)
  MATLAB Function3/1(theta) -> Mux3/1
  MATLAB Function1/1(y) -> ang velocity seesaw/1, "CoM6D ->  CoMXYZ2"/1
  inertial_seesaw/1 -> Selector3/1, Selector2/1
  Mux3/1 -> theta_seesaw/1

== system controller/Subsystem/w_H_root_link1 ==
  qj : Inport
  Constant2 : Constant  Value=eye(4)
  Constant6 : Constant  Value=eye(4)
  Inv\*1 : Product  Inputs=/*  Multiplication=Matrix(*)
  link : WBToolboxLibrary/wholeBodyModel/Kinematics/Forward Kinematics  frameName=link_name  robotName=WBT_robotName  localName=WBT_modelName  wbiFile=WBT_wbiFilename  wbiList=WBT_wbiList
  root_link : WBToolboxLibrary/wholeBodyModel/Kinematics/Forward Kinematics  frameName='root_link'  robotName=WBT_robotName  localName=WBT_modelName  wbiFile=WBT_wbiFilename  wbiList=WBT_wbiList
  link_H_root : Outport
  wires:
  Constant6/1 -> link/1
  Inv\*1/1 -> link_H_root/1  "link_H_root"
  link/1 -> Inv\*1/1
  Constant2/1 -> root_link/1
  qj/1 -> root_link/2, link/2
  root_link/1 -> Inv\*1/2

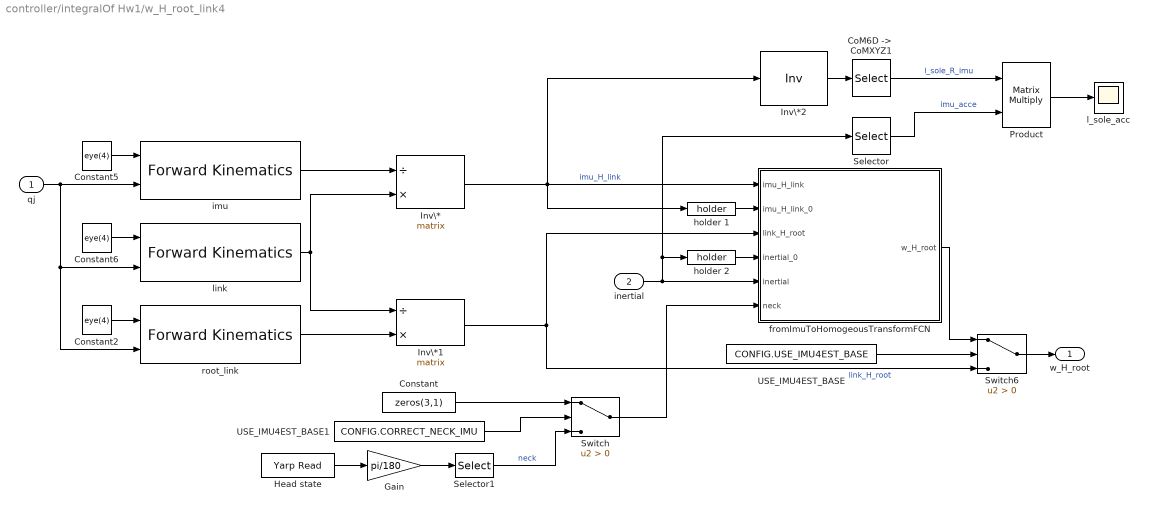
== system controller/integralOf Hw1/w_H_root_link4 ==
  qj : Inport
  inertial : Inport  Port=2
  "CoM6D ->  CoMXYZ1" : Selector  NumberOfDimensions=2  InputPortWidth=7  IndexOptions=Index vector (dialog),Index vector (dialog)  Indices=[1 2 3],[1 2 3]  OutputSizes=1,1
  Constant : Constant  Value=zeros(3,1)
  Constant2 : Constant  Value=eye(4)
  Constant5 : Constant  Value=eye(4)
  Constant6 : Constant  Value=eye(4)
  Gain : Gain  Gain=pi/180
  Head state : WBToolboxLibrary/Utilities/Yarp Read  portName=[WBT_robotName, '/head/state:o']  signalSize=6  blocking=off  timestamp=off  autoconnect=on  errorOnConnection=off
  Inv\* : Product  Inputs=/*  Multiplication=Matrix(*)
  Inv\*1 : Product  Inputs=/*  Multiplication=Matrix(*)
  Inv\*2 : Product  Inputs=/  Multiplication=Matrix(*)
  Product : Product  Multiplication=Matrix(*)
  Selector : Selector  InputPortWidth=12  IndexOptions=Index vector (dialog)  Indices=[4 5 6 ]  OutputSizes=1
  Selector1 : Selector  InputPortWidth=6  IndexOptions=Index vector (dialog)  Indices=[1:3]  OutputSizes=1
  Switch : Switch  Criteria=u2 > Threshold
  Switch6 : Switch  Criteria=u2 > Threshold
  USE_IMU4EST_BASE : Constant  Value=CONFIG.USE_IMU4EST_BASE
  USE_IMU4EST_BASE1 : Constant  Value=CONFIG.CORRECT_NECK_IMU
  fromImuToHomogeousTransformFCN : MATLAB Function  TreatAsAtomicUnit=on
  holder 1 : WBToolboxLibrary/Utilities/holder 
  holder 2 : WBToolboxLibrary/Utilities/holder 
  imu : WBToolboxLibrary/wholeBodyModel/Kinematics/Forward Kinematics  frameName='imu_frame'  robotName=WBT_robotName  localName=WBT_modelName  wbiFile=WBT_wbiFilename  wbiList=WBT_wbiList
  l_sole_acc : Scope
  link : WBToolboxLibrary/wholeBodyModel/Kinematics/Forward Kinematics  frameName=link_name  robotName=WBT_robotName  localName=WBT_modelName  wbiFile=WBT_wbiFilename  wbiList=WBT_wbiList
  root_link : WBToolboxLibrary/wholeBodyModel/Kinematics/Forward Kinematics  frameName='root_link'  robotName=WBT_robotName  localName=WBT_modelName  wbiFile=WBT_wbiFilename  wbiList=WBT_wbiList
  w_H_root : Outport
  wires:
  Constant5/1 -> imu/1
  Inv\*/1 -> Inv\*2/1, holder 1/1, fromImuToHomogeousTransformFCN/1(imu_H_link)  "imu_H_link"
  imu/1 -> Inv\*/1
  Constant6/1 -> link/1
  Inv\*1/1 -> Switch6/3, fromImuToHomogeousTransformFCN/3(link_H_root)  "link_H_root"
  link/1 -> Inv\*/2, Inv\*1/1
  inertial/1 -> Selector/1, holder 2/1, fromImuToHomogeousTransformFCN/5(inertial)
  Switch6/1 -> w_H_root/1
  USE_IMU4EST_BASE/1 -> Switch6/2
  fromImuToHomogeousTransformFCN/1(w_H_root) -> Switch6/1
  Constant2/1 -> root_link/1
  qj/1 -> root_link/2, link/2, imu/2
  root_link/1 -> Inv\*1/2
  holder 1/1 -> fromImuToHomogeousTransformFCN/2(imu_H_link_0)
  holder 2/1 -> fromImuToHomogeousTransformFCN/4(inertial_0)
  Inv\*2/1 -> "CoM6D ->  CoMXYZ1"/1
  "CoM6D ->  CoMXYZ1"/1 -> Product/1  "l_sole_R_imu"
  Selector/1 -> Product/2  "imu_acce"
  Product/1 -> l_sole_acc/1
  Head state/1 -> Gain/1
  Selector1/1 -> Switch/3  "neck"
  Constant/1 -> Switch/1
  USE_IMU4EST_BASE1/1 -> Switch/2
  Switch/1 -> fromImuToHomogeousTransformFCN/6(neck)
  Gain/1 -> Selector1/1

== system controller/synchronizer/GAZEBO_SYNCHRONIZER ==
  Enable : EnablePort
  Simulator Synchronizer : WBToolboxLibrary/Utilities/Simulator Synchronizer  period=CONFIG.TS  serverPortName='/clock/rpc'  clientPortName='/WBT_synchronizer/rpc:o'

== system controller/synchronizer/REAL_TIME_SYNC ==
  Enable : EnablePort
  Real Time Synchronizer : WBToolboxLibrary/Utilities/Real Time Synchronizer  period=CONFIG.TS

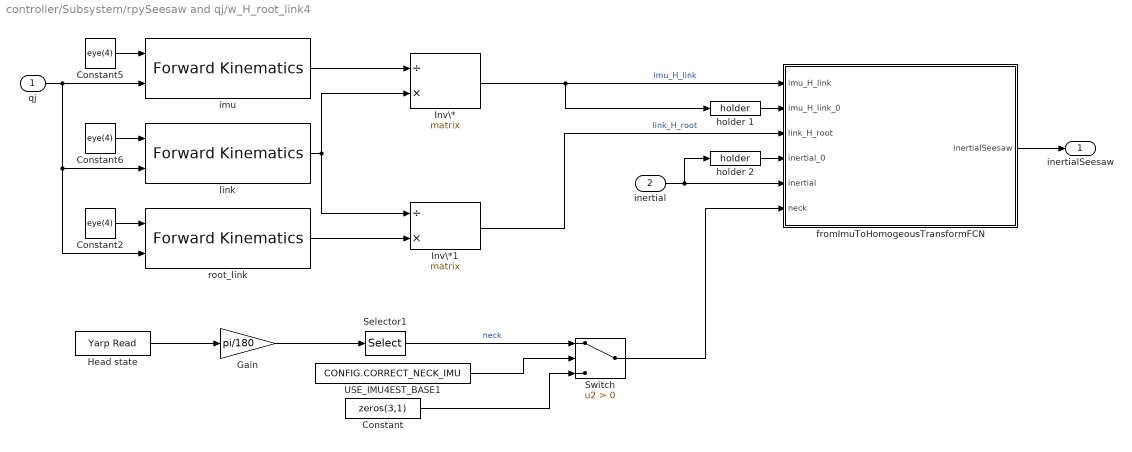
== system controller/Subsystem/rpySeesaw and qj/w_H_root_link4 ==
  qj : Inport
  inertial : Inport  Port=2
  Constant : Constant  Value=zeros(3,1)
  Constant2 : Constant  Value=eye(4)
  Constant5 : Constant  Value=eye(4)
  Constant6 : Constant  Value=eye(4)
  Gain : Gain  Gain=pi/180
  Head state : WBToolboxLibrary/Utilities/Yarp Read  portName=PORTS.NECK  signalSize=6  blocking=off  timestamp=off  autoconnect=on  errorOnConnection=on
  Inv\* : Product  Inputs=/*  Multiplication=Matrix(*)
  Inv\*1 : Product  Inputs=/*  Multiplication=Matrix(*)
  Selector1 : Selector  InputPortWidth=6  IndexOptions=Index vector (dialog)  Indices=[1:3]  OutputSizes=1
  Switch : Switch  Criteria=u2 > Threshold
  USE_IMU4EST_BASE1 : Constant  Value=CONFIG.CORRECT_NECK_IMU
  fromImuToHomogeousTransformFCN : MATLAB Function  TreatAsAtomicUnit=on
  holder 1 : WBToolboxLibrary/Utilities/holder 
  holder 2 : WBToolboxLibrary/Utilities/holder 
  imu : WBToolboxLibrary/wholeBodyModel/Kinematics/Forward Kinematics  frameName='imu_frame'  robotName=WBT_robotName  localName=WBT_modelName  wbiFile=WBT_wbiFilename  wbiList=WBT_wbiList
  link : WBToolboxLibrary/wholeBodyModel/Kinematics/Forward Kinematics  frameName=link_name  robotName=WBT_robotName  localName=WBT_modelName  wbiFile=WBT_wbiFilename  wbiList=WBT_wbiList
  root_link : WBToolboxLibrary/wholeBodyModel/Kinematics/Forward Kinematics  frameName='root_link'  robotName=WBT_robotName  localName=WBT_modelName  wbiFile=WBT_wbiFilename  wbiList=WBT_wbiList
  inertialSeesaw : Outport
  wires:
  Constant5/1 -> imu/1
  Inv\*/1 -> holder 1/1, fromImuToHomogeousTransformFCN/1(imu_H_link)  "imu_H_link"
  imu/1 -> Inv\*/1
  Constant6/1 -> link/1
  Inv\*1/1 -> fromImuToHomogeousTransformFCN/3(link_H_root)  "link_H_root"
  link/1 -> Inv\*/2, Inv\*1/1
  inertial/1 -> holder 2/1, fromImuToHomogeousTransformFCN/5(inertial)
  fromImuToHomogeousTransformFCN/1(inertialSeesaw) -> inertialSeesaw/1
  Constant2/1 -> root_link/1
  qj/1 -> root_link/2, link/2, imu/2
  root_link/1 -> Inv\*1/2
  holder 1/1 -> fromImuToHomogeousTransformFCN/2(imu_H_link_0)
  holder 2/1 -> fromImuToHomogeousTransformFCN/4(inertial_0)
  Head state/1 -> Gain/1
  Selector1/1 -> Switch/1  "neck"
  USE_IMU4EST_BASE1/1 -> Switch/2
  Switch/1 -> fromImuToHomogeousTransformFCN/6(neck)
  Gain/1 -> Selector1/1
  Constant/1 -> Switch/3

== matlab function balancingControlSeeSawFCN ==
  data: comError output double; fNoQp output double; f_HDot output double; NA output double; t input double; x0 input double; x input double; ConstraintsMatrix input double; bVectorConstraints input double; gain parameter double; reg parameter double; xcomRef input double; qdesRef input double; seesaw parameter double; ROBOT_DOF input double; J input double; J_CoM input double; JdotNu input double; M input double; genBiasForces input double; w_p_com input double; w_H_l_sole input double; w_H_r_sole input double; H input double; intHw input double; CONFIG parameter double; tauModel output double; Sigmaf_HDot output double; SigmaNA output double; HessianMatrixQP2Feet output double; gradientQP2Feet output double; ConstraintsMatrixQP2Feet output double; bVectorConstraintsQp2Feet output double; psat output double; yCoM_des output double
function [comError,fNoQp,f_HDot,NA,tauModel,Sigmaf_HDot,SigmaNA,...
          HessianMatrixQP2Feet,gradientQP2Feet,ConstraintsMatrixQP2Feet,bVectorConstraintsQp2Feet, psat,yCoM_des] = ...
          balancingControlSeeSawFCN(t,x0,x,ConstraintsMatrix,bVectorConstraints, gain, reg, ...
                                    xcomRef, qdesRef, seesaw, ROBOT_DOF,...
                                    J, J_CoM, JdotNu, M, genBiasForces, w_p_com, w_H_l_sole, w_H_r_sole,H,intHw,CONFIG)
%#codegen
    robot                              = struct;

    robot.M                            = M;
    robot.J                            = J;
    robot.JdotNu                       = JdotNu;
    robot.genBiasForces                = genBiasForces;
    robot.fwdkin.w_p_com               = w_p_com;
    robot.fwdkin.w_H_l_sole            = w_H_l_sole;
    robot.fwdkin.w_H_r_sole            = w_H_r_sole;

    robot.lFootDistanceCenter          = seesaw.lFootDistanceCenter;
    robot.rFootDistanceCenter          = seesaw.rFootDistanceCenter;

    controlParams.gain                 = gain;
    controlParams.references.qDes      = qdesRef;
    controlParams.references.xcomDes   = xcomRef(:,1);
    controlParams.references.DxcomDes  = xcomRef(:,2);
    controlParams.references.DDxcomDes = xcomRef(:,3);

    model = struct('robot', robot, 'seesaw', seesaw);

    [comError,fNoQp,f_HDot,NA,tauModel,Sigmaf_HDot,SigmaNA,...
              HessianMatrixQP2Feet,gradientQP2Feet,ConstraintsMatrixQP2Feet,bVectorConstraintsQp2Feet, psat,yCoM_des] = ...
              balancingControlSeeSaw(t, x,ConstraintsMatrix,bVectorConstraints,J_CoM,H,intHw,controlParams, model, robot,reg,CONFIG,gain,ROBOT_DOF);

end

== matlab function Subsystem/MATLAB Function ==
  data: Qs output double; w_H_l_sole output double; inertialSeesaw input double; seesaw parameter double
function [Qs,w_H_l_sole] = computeRotTransFromLsole2WorldFCN(inertialSeesaw,seesaw)
%#codegen

    % Compute w_H_l_sole
    [Qs,w_H_l_sole] = computeRotTransFromLsole2World(inertialSeesaw,seesaw);

end

== matlab function CoM and qj at t = 0/trajectoryGeneratorCoM ==
  data: desired_x_dx_ddx_CoM output double; xCom0 input double; t input double; referenceParams input double; x2D input double; directionOfOscillation input double; noOscillationTime input double
function desired_x_dx_ddx_CoM   = fcn(xCom0,t,referenceParams,x2D,directionOfOscillation,noOscillationTime)
%#codegen

if t > noOscillationTime
    A = referenceParams(1);
else
    A = 0;
end

f          =  referenceParams(2);

xcomDes    =  xCom0 + A*sin(2*pi*f*t)*directionOfOscillation;
% xcomDes(1) =  xcomDes(1) + 0.01;
xDcomDes   =  A*2*pi*f*cos(2*pi*f*t)*directionOfOscillation;
xDDcomDes  = -A*(2*pi*f)^2*sin(2*pi*f*t)*directionOfOscillation;
xcomDes(2) =  x2D + xCom0(2);

desired_x_dx_ddx_CoM = [xcomDes;xDcomDes;xDDcomDes];

end

== matlab function Subsystem/baseVel/evaluateBaseVelocity ==
  data: w_v_base output double; J_l_sole input double; w_H_l_sole input double; dq_j input double; s_omega_s input double; model parameter double
function w_v_base  = computeBaseVelocityFCN(J_l_sole, w_H_l_sole,dq_j, s_omega_s, model)
%#codegen

    w_v_base  = computeBaseVelocity(J_l_sole, w_H_l_sole,dq_j, s_omega_s, model);

end

== matlab function Subsystem/Visualize hom transf1/MATLAB Function ==
  data: R input double; rollPitchYaw output double
function rollPitchYaw = buildHomogenousTranformation(R)
%#codegen

rollPitchYaw = rollPitchYawFromRotation(R);

rollPitchYaw = rollPitchYaw*180/pi;

== matlab function Subsystem/Visualize hom transf2/MATLAB Function ==
  data: R input double; rollPitchYaw output double
function rollPitchYaw = buildHomogenousTranformation(R)
%#codegen

rollPitchYaw = rollPitchYawFromRotation(R);

rollPitchYaw = rollPitchYaw*180/pi;

== matlab function Subsystem/rpySeesaw and qj/w_H_root_link4/fromImuToHomogeousTransformFCN ==
  data: imu_H_link input double; imu_H_link_0 input double; link_H_root input double; inertial_0 input double; inertial input double; neck input double; inertialSeesaw output double; CONFIG parameter double
function inertialSeesaw = fromBaseToWorldWithImuFCN(imu_H_link,imu_H_link_0,link_H_root,inertial_0,inertial,neck,CONFIG)
%#codegen

 [~,w_R_link] = fromBaseToWorldWithImuSeesaw(imu_H_link,imu_H_link_0,link_H_root,inertial_0,inertial,neck,CONFIG);
 
 rollPitchYaw_link   = rollPitchYawFromRotation(w_R_link);

 s_omega_seesaw = zeros(3,1);
 
 inertialSeesaw = [rollPitchYaw_link*(180/pi);zeros(3,1); s_omega_seesaw; zeros(3,1)];

== matlab function Subsystem/seesaw IMU/MATLAB Function1 ==
  data: u input double; y output double
function y = rotate(u)

y = rotx(pi)*rotz(-44/180*pi)*u;

== matlab function Subsystem/seesaw IMU/MATLAB Function2 ==
  data: u input double; y output double
function y = rotate(u)

y = rotx(pi)*rotz(-44/180*pi)*u;

end

== matlab function Subsystem/seesaw IMU/MATLAB Function3 ==
  data: acc input double; theta output double
function theta = arctangent(acc)

theta = atan2(acc(2),acc(3))*180/pi;

== matlab function integralOf Hw1/MATLAB Function ==
  data: qjErr input double; JL input double; JR input double; vbEquivalent output double; reg parameter double; activeFeetConstraints input double
 function vbEquivalent = generateReferencesForH(qjErr,JL,JR,reg,activeFeetConstraints)
%#codegen
if activeFeetConstraints(1) == 1
    
pinvJb             = (JL(:,1:6)'*JL(:,1:6) + reg.pinvDampVb*eye(6))\JL(:,1:6)';
vbEquivalent       = -pinvJb*JL(:,7:end)*qjErr;
else
    
pinvJb             = (JR(:,1:6)'*JR(:,1:6) + reg.pinvDampVb*eye(6))\JR(:,1:6)';
vbEquivalent       = -pinvJb*JR(:,7:end)*qjErr;
end
    
end

== matlab function Subsystem/Visualize hom transf5/MATLAB Function ==
  data: R input double; rollPitchYaw output double
function rollPitchYaw = buildHomogenousTranformation(R)
%#codegen

rollPitchYaw = rollPitchYawFromRotation(R);

rollPitchYaw = rollPitchYaw*180/pi;

== matlab function integralOf Hw1/w_H_root_link4/fromImuToHomogeousTransformFCN ==
  data: imu_H_link input double; imu_H_link_0 input double; link_H_root input double; inertial_0 input double; inertial input double; neck input double; w_H_root output double; CONFIG parameter double
function w_H_root = fromBaseToWorldWithImuFCN(imu_H_link,imu_H_link_0,link_H_root,inertial_0,inertial,neck,CONFIG)
%#codegen
w_H_root = fromBaseToWorldWithImu(imu_H_link,imu_H_link_0,link_H_root,inertial_0,inertial,neck,CONFIG);
